simulink model "Project5"  (R2023b)
settings: Solver=VariableStepAuto  StartTime=0.0  StopTime=Sim_Time  RelTol=1e-3
values from neighbouring files (symbols this model uses):
  Cn = 2.3*3600    (= 8280)    [project5_me.m]
  I = 2.3    [project5_me.m]
  OCV = Data(:,2)    [project5_me.m]
  R_discharge = Data(:,4)    [project5_me.m]
  SoC = Data(:,1)    [project5_me.m]
settings Model: Creator=91753  LastModifiedBy=91753

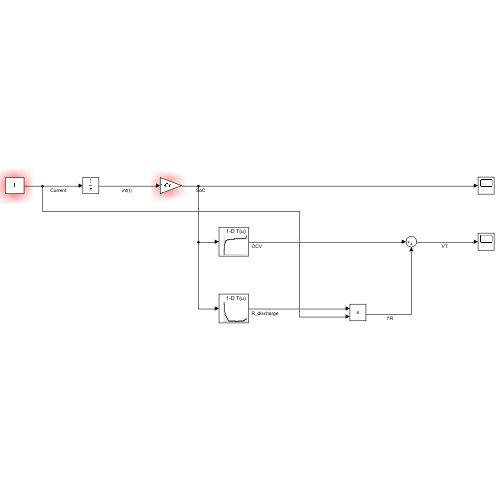
[thumbnail: Simulink's stored preview of the top-level diagram]
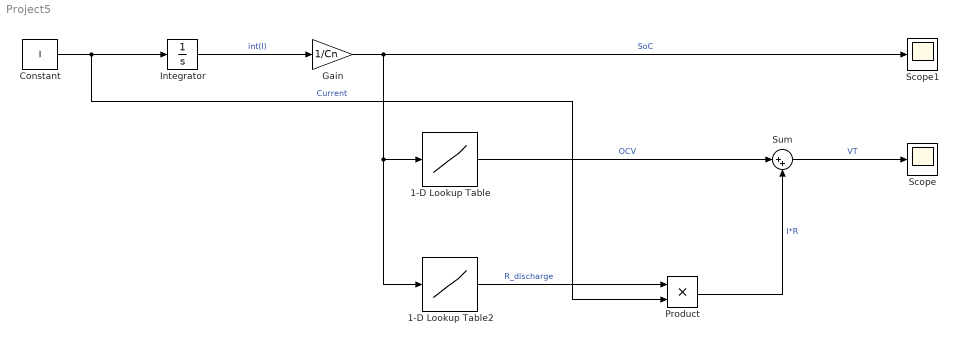
== system Project5 ==
  1-D Lookup Table : Lookup_n-D  NumberOfTableDimensions=1  BreakpointsForDimension1=SoC  Table=OCV  InternalRulePriority=Speed  RndMeth=Simplest
  1-D Lookup Table2 : Lookup_n-D  NumberOfTableDimensions=1  BreakpointsForDimension1=SoC  Table=R_discharge  InternalRulePriority=Speed  RndMeth=Simplest
  Constant : Constant  Value=I
  Gain : Gain  Gain=1/Cn
  Integrator : Integrator
  Product : Product
  Scope : Scope
  Scope1 : Scope
  Sum : Sum  Inputs=|++
  wires:
  Constant/1 -> Product/2, Integrator/1  "Current"
  Integrator/1 -> Gain/1  "int(I)"
  Gain/1 -> Scope1/1, 1-D Lookup Table2/1, 1-D Lookup Table/1  "SoC"
  1-D Lookup Table/1 -> Sum/1  "OCV"
  1-D Lookup Table2/1 -> Product/1  "R_discharge"
  Product/1 -> Sum/2  "I*R"
  Sum/1 -> Scope/1  "VT"
